simulink model "Lab_2_sim"  (R2017a)
settings: Solver=VariableStepAuto  StartTime=0.0  StopTime=1.0  RelTol=1e-3
values from neighbouring files (symbols this model uses):
  alpha = 26.66    [Lab_2.m]
  alphap = 32.7345    [Lab_2.m]
  beta = 133.33    [Lab_2.m]
  K = (alphap/2)^2/beta    (= 2.00920177426)    [Lab_2.m]
  T = 0.001    [Lab_2.m]
settings Model: Creator=njohnson  LastModifiedBy=njohnson

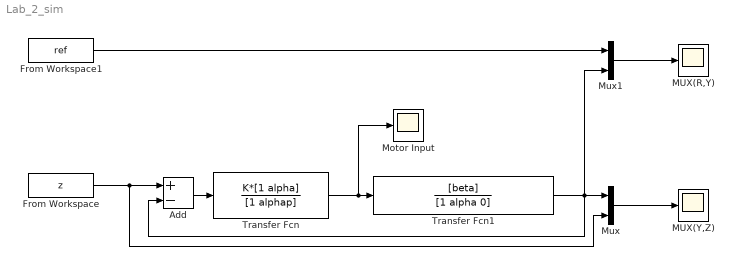
== system Lab_2_sim ==
  Add : Sum  Inputs=+-
  From Workspace : FromWorkspace  VariableName=z  SampleTime=T  OutputAfterFinalValue=Holding final value
  From Workspace1 : FromWorkspace  VariableName=ref  SampleTime=T  OutputAfterFinalValue=Holding final value
  "MUX(R,Y) " : Scope
  "MUX(Y,Z) " : Scope
  "Motor Input " : Scope
  Mux : Mux  Inputs=2
  Mux1 : Mux  Inputs=2
  Transfer Fcn : TransferFcn  Numerator=K*[1 alpha]  Denominator=[1 alphap]
  Transfer Fcn1 : TransferFcn  Numerator=[beta]  Denominator=[1 alpha 0]
  wires:
  Add/1 -> Transfer Fcn/1
  Transfer Fcn/1 -> "Motor Input "/1, Transfer Fcn1/1
  From Workspace/1 -> Add/1, Mux/2
  Transfer Fcn1/1 -> Add/2, Mux1/2, Mux/1
  From Workspace1/1 -> Mux1/1
  Mux1/1 -> "MUX(R,Y) "/1
  Mux/1 -> "MUX(Y,Z) "/1
